simulink model "ld3_fixed_point2"  (R2017b)
settings: Solver=FixedStepDiscrete  StartTime=0.01  StopTime=0.02  RelTol=1e-3
settings Model: Creator=Imants  LastModifiedBy=Imants
settings OptimizationCC: BlockReduction=off  ConditionallyExecuteInputs=off
settings DebuggingCC: SingleTaskRateTransMsg=error  SFTemporalDelaySmallerThanSampleTimeDiag=none

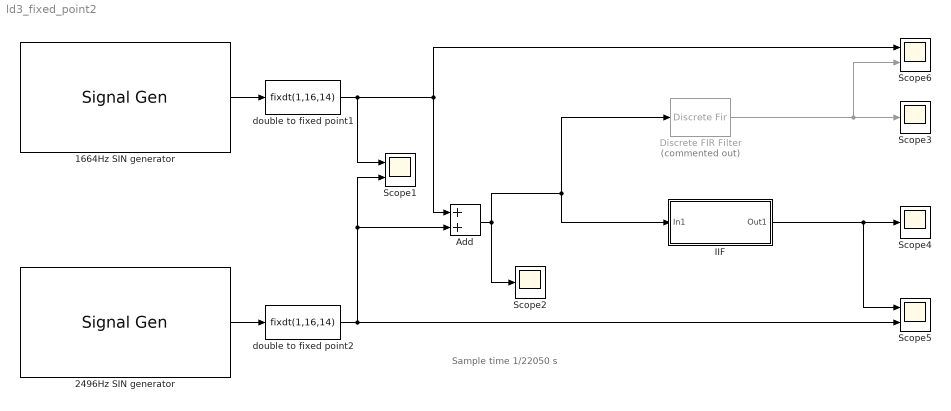
== system ld3_fixed_point2 ==
  note: Sample time 1/22050 s
  1664Hz SIN generator : SignalGenerator  Frequency=1664
  2496Hz SIN generator : SignalGenerator  Frequency=2496
  Add : Sum
  "Discrete FIR Filter " : DiscreteFir  Commented=on  Coefficients="[-0.0073   -0.0071   -0.0059   -0.0024    0.0040    0.0133    0.0231    0.0301    0.0302    0.0207    0.0014   -0.0242   -0.0498 -0.0677   -0.0713   -0.0571   -0.0269    0.0129    0.0525    0.0814    0.0921    0.0814    0.0525    0.0129   -0.0269   -0.0571 -0.0713   -0.0677   -0.0498   -0.0242    0.0014    0.0207    0.0302    0.0301    0.0231    0.0133    0.0040   -0.0024   -0.0059 -0.0071   -0.0073]"  CoefDataTypeStr=fixdt(1,16,14)  ProductDataTypeStr=fixdt(1,16,14)  AccumDataTypeStr=fixdt(1,16,14)  OutDataTypeStr=fixdt(1,16,14)
  IIF : Subsystem
  Scope1 : Scope  NumInputPorts=2
  Scope2 : Scope
  Scope3 : Scope
  Scope4 : Scope
  Scope5 : Scope  NumInputPorts=2
  Scope6 : Scope  NumInputPorts=2
  double to fixed point1 : DataTypeConversion  OutDataTypeStr=fixdt(1,16,14)
  double to fixed point2 : DataTypeConversion  OutDataTypeStr=fixdt(1,16,14)
  wires:
  2496Hz SIN generator/1 -> double to fixed point2/1
  1664Hz SIN generator/1 -> double to fixed point1/1
  double to fixed point1/1 -> Scope1/1, Add/1, Scope6/1
  double to fixed point2/1 -> Scope5/2, Add/2, Scope1/2
  IIF/1(Out1) -> Scope5/1, Scope4/1
  "Discrete FIR Filter "/1 -> Scope6/2, Scope3/1
  Add/1 -> Scope2/1, "Discrete FIR Filter "/1, IIF/1(In1)

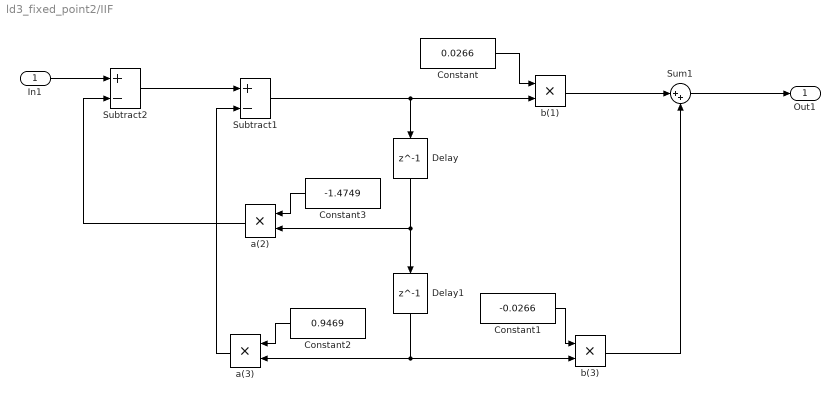
== system ld3_fixed_point2/IIF ==
  In1 : Inport  OutDataTypeStr=fixdt(1,16,14)
  Constant : Constant  Value=0.0266  OutDataTypeStr=fixdt(0,16,21)
  Constant1 : Constant  Value=-0.0266  OutDataTypeStr=fixdt(1,16,20)
  Constant2 : Constant  Value=0.9469  OutDataTypeStr=fixdt(0,16,16)
  Constant3 : Constant  Value=-1.4749  OutDataTypeStr=fixdt(1,16,14)
  Delay : Delay  DelayLength=1  InitialCondition=0
  Delay1 : Delay  DelayLength=1  InitialCondition=0
  Subtract1 : Sum  Inputs=+-  OutDataTypeStr=fixdt(1,16,9)
  Subtract2 : Sum  Inputs=+-  OutDataTypeStr=fixdt(1,16,9)
  Sum1 : Sum  Inputs=|++  OutDataTypeStr=fixdt(1,16,14)
  a(2) : Product  OutDataTypeStr=fixdt(1,16,9)
  a(3) : Product  OutDataTypeStr=fixdt(1,16,10)
  b(1) : Product  OutDataTypeStr=fixdt(1,16,15)
  b(3) : Product  OutDataTypeStr=fixdt(1,16,15)
  Out1 : Outport
  wires:
  In1/1 -> Subtract2/1
  Subtract2/1 -> Subtract1/1
  Subtract1/1 -> Delay/1, b(1)/2
  Delay/1 -> a(2)/2, Delay1/1
  Delay1/1 -> a(3)/2, b(3)/2
  Sum1/1 -> Out1/1
  Constant/1 -> b(1)/1
  b(1)/1 -> Sum1/1
  Constant1/1 -> b(3)/1
  b(3)/1 -> Sum1/2
  Constant2/1 -> a(3)/1
  a(3)/1 -> Subtract1/2
  Constant3/1 -> a(2)/1
  a(2)/1 -> Subtract2/2
